simulink model "KvadroModel"  (R2013a)
settings: Solver=ode45  StartTime=0.0  StopTime=60  RelTol=1e-3
libraries: aerolibfltsims x2, vrlib x1, aerolib6dof2 x1, aerolibutil x1
settings Model: Creator=Mirag_000  LastModifiedBy=Mirag_000
settings DataIOCC: SignalLoggingSaveFormat=ModelDataLogs
settings DebuggingCC: MultiTaskDSMMsg=warning  MultiTaskCondExecSysMsg=none  StrictBusMsg=None
settings RTWCC: IncludeERTFirstTime=on

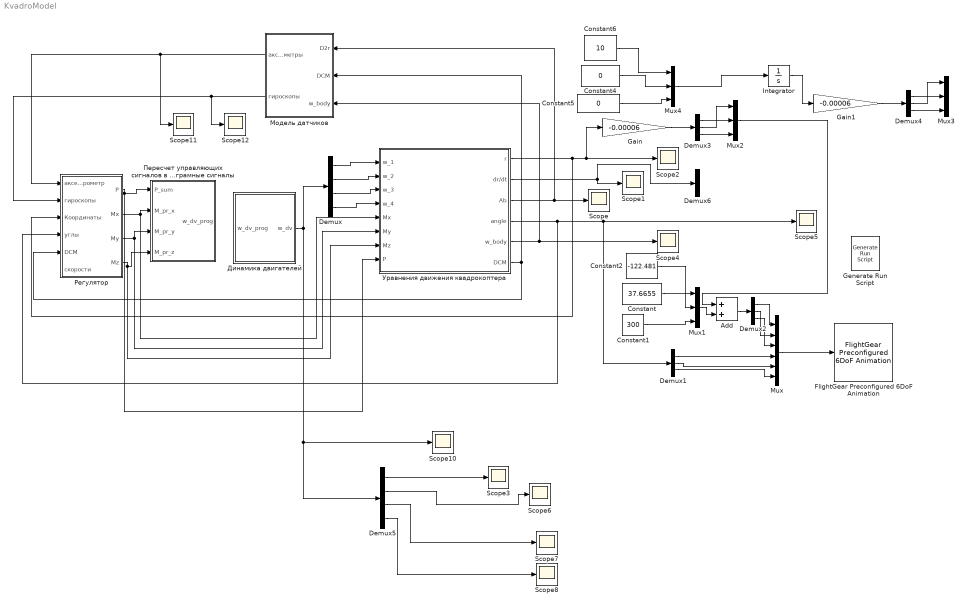
== system KvadroModel ==
  Add : Sum
  Constant : Constant  Value=37.6655
  Constant1 : Constant  Value=300
  Constant2 : Constant  Value=-122.481
  Constant4 : Constant  Value=0
  Constant5 : Constant  Value=0
  Constant6 : Constant  Value=10
  Demux : Demux
  Demux{1..4,6} (5 alike) : Demux  Outputs=3
  Demux5 : Demux
  FlightGear Preconfigured 6DoF Animation : aerolibfltsims/FlightGear Preconfigured 6DoF Animation  xFlightGearVersion=v2.8  DestinationIpAddress=127.0.0.1  DestinationPort=5502  SampleTime=1/30
  Gain : Gain  Gain=-0.00006
  Gain1 : Gain  Gain=-0.00006
  Generate Run Script : aerolibfltsims/Generate Run Script  OutputFileName=I:\Program Files\FlightGear\runfg.bat  FlightGearBaseDirectory=I:\Program Files\FlightGear  GeometryModelName=arducopter  DestinationPort=5502  OriginAddress=127.0.0.1  OriginPort=5505  LocalAddress=127.0.0.1  AirportId=KSFO  RunwayId=10L  InitialAltitude=7224  InitialHeading=113  OffsetDistance=4.72  OffsetAzimuth=0  GenerateFile=off  Architecture=Default  dataFlow=Send
  Integrator : Integrator
  Mux : Mux  Inputs=6
  Mux{1..4} (4 alike) : Mux  Inputs=3
  Scope{,1..8,10..12} (12 alike) : Scope
      Scope settings: TimeRange=60  YMin=-10  YMax=25
      Scope1 settings: YMin=-40  YMax=15  SaveName=ScopeData4
      Scope10 settings: YMin=1.5  YMax=3.75  SaveName=ScopeData12
      Scope11 settings: SaveName=ScopeData14
      Scope12 settings: SaveName=ScopeData15
      Scope2 settings: YMin=-80  YMax=90  SaveName=ScopeData5
      Scope3 settings: YMin=5.745  YMax=5.805  SaveName=ScopeData37
      Scope4 settings: YMin=-0.2  YMax=0.025  SaveName=ScopeData6
      Scope5 settings: YMin=-1.4  YMax=0.2  SaveName=ScopeData7
      Scope6 settings: YMin=5.73  YMax=5.82  SaveName=ScopeData38
      Scope7 settings: YMin=1.6525  YMax=1.675  SaveName=ScopeData46
      Scope8 settings: YMin=1.5  YMax=3.75  SaveName=ScopeData47
  Динамика двигателей : Subsystem
  Модель датчиков : Subsystem
  Пересчет управляющих сигналов в програмные сигналы : Subsystem
  Регулятор : Subsystem
  Уравнения движения квадрокоптера : Subsystem
  wires:
  Уравнения движения квадрокоптера/3(Ab) -> Scope/1, Модель датчиков/1(D2r)
  Уравнения движения квадрокоптера/2(dr/dt) -> Scope1/1, Demux6/1
  Уравнения движения квадрокоптера/1(r) -> Регулятор/3(Координаты), Gain/1, Scope2/1
  Уравнения движения квадрокоптера/5(w_body) -> Scope4/1, Модель датчиков/3(w_body)
  Уравнения движения квадрокоптера/4(angle) -> Регулятор/4(углы), Demux1/1, Scope5/1
  Demux/1 -> Уравнения движения квадрокоптера/1(w_1)
  Demux/2 -> Уравнения движения квадрокоптера/2(w_2)
  Demux/3 -> Уравнения движения квадрокоптера/3(w_3)
  Demux/4 -> Уравнения движения квадрокоптера/4(w_4)
  Динамика двигателей/1(w_dv) -> Demux5/1, Scope10/1, Demux/1
  Регулятор/1(P) -> Пересчет управляющих сигналов в програмные сигналы/1(P_sum), Уравнения движения квадрокоптера/8(P)
  Модель датчиков/1(акселерометры) -> Scope11/1, Регулятор/1(акселерометр)
  Модель датчиков/2(гироскопы) -> Scope12/1, Регулятор/2(гироскопы)
  Регулятор/2(Mx) -> Уравнения движения квадрокоптера/5(Mx), Пересчет управляющих сигналов в програмные сигналы/2(M_pr_x)
  Регулятор/3(My) -> Уравнения движения квадрокоптера/6(My), Пересчет управляющих сигналов в програмные сигналы/3(M_pr_y)
  Уравнения движения квадрокоптера/6("DCM ") -> Регулятор/5(DCM), Модель датчиков/2(DCM)
  Demux1/3 -> Mux/6
  Demux1/2 -> Mux/5
  Demux1/1 -> Mux/4
  Mux/1 -> FlightGear Preconfigured 6DoF Animation/1
  Constant2/1 -> Mux1/1
  Constant/1 -> Mux1/2
  Constant1/1 -> Mux1/3
  Mux1/1 -> Add/2
  Add/1 -> Demux2/1
  Demux2/3 -> Mux/3
  Demux2/2 -> Mux/2
  Demux2/1 -> Mux/1
  Gain/1 -> Demux3/1
  Demux3/3 -> Mux2/3
  Gain1/1 -> Demux4/1
  Demux4/3 -> Mux3/3
  Demux4/2 -> Mux3/1
  Demux4/1 -> Mux3/2
  Integrator/1 -> Gain1/1
  Constant5/1 -> Mux4/3
  Mux4/1 -> Integrator/1
  Constant6/1 -> Mux4/1
  Constant4/1 -> Mux4/2
  Mux2/1 -> Add/1
  Demux3/1 -> Mux2/2
  Demux3/2 -> Mux2/1
  Demux5/1 -> Scope3/1
  Demux5/2 -> Scope6/1
  Demux5/3 -> Scope7/1
  Demux5/4 -> Scope8/1
  Регулятор/4(Mz) -> Уравнения движения квадрокоптера/7(Mz), Пересчет управляющих сигналов в програмные сигналы/4(M_pr_z)

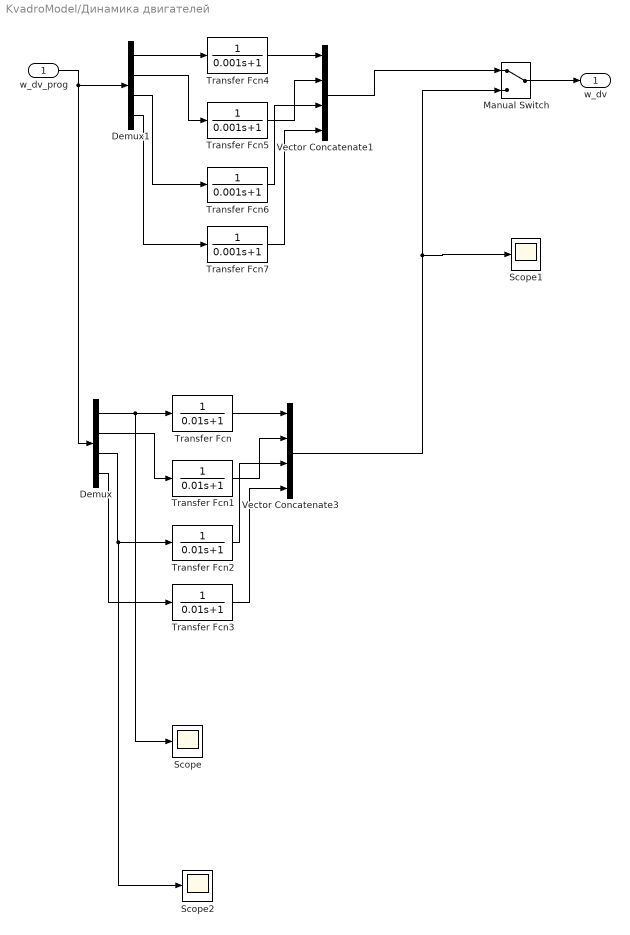
== system KvadroModel/Динамика двигателей ==
  w_dv_prog : Inport
  Demux : Demux
  Demux1 : Demux
  Manual Switch : ManualSwitch
  Scope : Scope
      settings: TimeRange=60  YMin=1.6595  YMax=1.668  SaveName=ScopeData39
  Scope1 : Scope
      settings: YMin=1.655  YMax=1.675  SaveName=ScopeData42
  Scope2 : Scope
      settings: YMin=1.6595  YMax=1.668  SaveName=ScopeData50
  Transfer Fcn{,1..3} (4 alike) : TransferFcn  Denominator=[0.01 1]
  Transfer Fcn{4..7} (4 alike) : TransferFcn  Denominator=[0.001 1]
  Vector Concatenate1 : Concatenate  NumInputs=4
  Vector Concatenate3 : Concatenate  NumInputs=4
  w_dv : Outport
  wires:
  Transfer Fcn1/1 -> Vector Concatenate3/2
  Transfer Fcn2/1 -> Vector Concatenate3/3
  Transfer Fcn3/1 -> Vector Concatenate3/4
  Vector Concatenate3/1 -> Scope1/1, Manual Switch/2
  Demux/1 -> Scope/1, Transfer Fcn/1
  Transfer Fcn/1 -> Vector Concatenate3/1
  Demux/2 -> Transfer Fcn1/1
  Demux/3 -> Scope2/1, Transfer Fcn2/1
  Demux/4 -> Transfer Fcn3/1
  Manual Switch/1 -> w_dv/1
  w_dv_prog/1 -> Demux/1, Demux1/1
  Transfer Fcn5/1 -> Vector Concatenate1/2
  Transfer Fcn6/1 -> Vector Concatenate1/3
  Transfer Fcn7/1 -> Vector Concatenate1/4
  Demux1/1 -> Transfer Fcn4/1
  Transfer Fcn4/1 -> Vector Concatenate1/1
  Demux1/2 -> Transfer Fcn5/1
  Demux1/3 -> Transfer Fcn6/1
  Demux1/4 -> Transfer Fcn7/1
  Vector Concatenate1/1 -> Manual Switch/1

== system KvadroModel/Модель датчиков ==
  D2r : Inport
  DCM : Inport  Port=2
  w_body : Inport  Port=3
  Add : Sum  Inputs=+-
  Constant : Constant  Value=[0 0 -9.81]
  Product : Product  Multiplication=Matrix(*)  RndMeth=Zero
  Scope : Scope
      settings: SaveName=ScopeData24
  акселерометры : Outport
  гироскопы : Outport  Port=2
  wires:
  D2r/1 -> Add/1
  w_body/1 -> Scope/1, гироскопы/1
  DCM/1 -> Product/1
  Constant/1 -> Product/2
  Product/1 -> Add/2
  Add/1 -> акселерометры/1

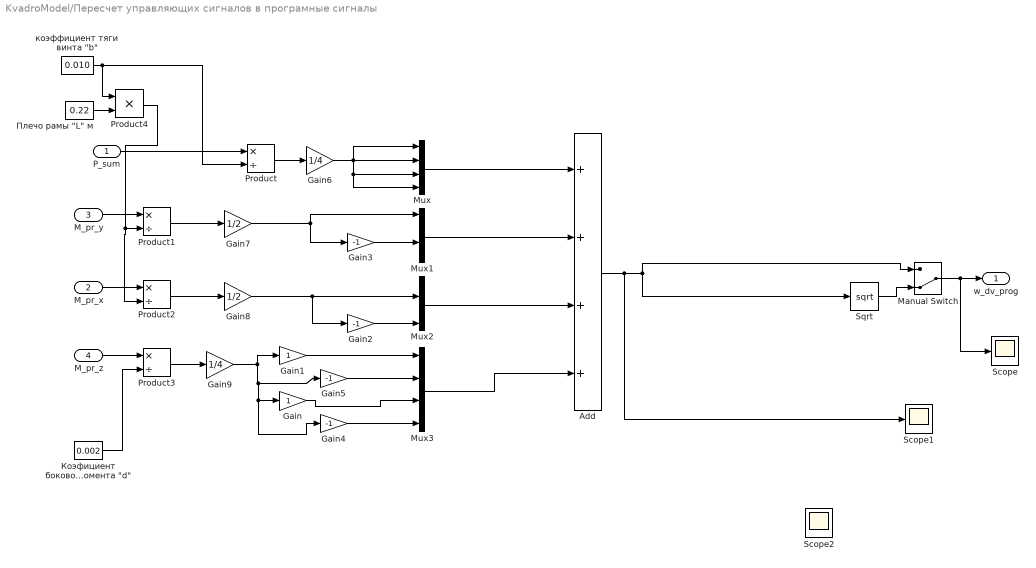
== system KvadroModel/Пересчет управляющих сигналов в програмные сигналы ==
  P_sum : Inport
  M_pr_x : Inport  Port=2
  M_pr_y : Inport  Port=3
  M_pr_z : Inport  Port=4
  Add : Sum  Inputs=++++
  Gain : Gain
  Gain1 : Gain
  Gain{2..5} (4 alike) : Gain  Gain=-1
  Gain6 : Gain  Gain=1/4
  Gain7 : Gain  Gain=1/2
  Gain8 : Gain  Gain=1/2
  Gain9 : Gain  Gain=1/4
  Manual Switch : ManualSwitch  CurrentSetting=0
  Mux{,1..3} (4 alike) : Mux
  Product{,1..3} (4 alike) : Product  Inputs=*/
  Product4 : Product
  Scope : Scope
      settings: YMin=1.6575  YMax=1.6775  SaveName=ScopeData20
  Scope1 : Scope
      settings: YMin=60  YMax=180  SaveName=ScopeData34
  Scope2 : Scope
      settings: YMin=0.07  YMax=0.1025  SaveName=ScopeData44
  Sqrt : Sqrt  SaturateOnIntegerOverflow=on
  "Коэфициент бокового момента \"d\"" : Constant  Value=0.002
  "Плечо рамы \"L\" м" : Constant  Value=0.22
  "коэффициент тяги винта \"b\"" : Constant  Value=0.010
  w_dv_prog : Outport
  wires:
  Gain/1 -> Mux3/3
  Gain1/1 -> Mux3/1
  Product3/1 -> Gain9/1
  Product2/1 -> Gain8/1
  Gain2/1 -> Mux2/4
  Gain3/1 -> Mux1/3
  Product1/1 -> Gain7/1
  Product/1 -> Gain6/1
  Mux2/1 -> Add/3
  Mux1/1 -> Add/2
  Mux/1 -> Add/1
  Mux3/1 -> Add/4
  Gain5/1 -> Mux3/2
  Gain4/1 -> Mux3/4
  Manual Switch/1 -> w_dv_prog/1, Scope/1
  Sqrt/1 -> Manual Switch/2
  Add/1 -> Scope1/1, Manual Switch/1, Sqrt/1
  P_sum/1 -> Product/1
  M_pr_y/1 -> Product1/1
  M_pr_x/1 -> Product2/1
  M_pr_z/1 -> Product3/1
  "Коэфициент бокового момента \"d\""/1 -> Product3/2
  "Плечо рамы \"L\" м"/1 -> Product4/2
  "коэффициент тяги винта \"b\""/1 -> Product/2, Product4/1
  Product4/1 -> Product2/2, Product1/2
  Gain6/1 -> Mux/4, Mux/3, Mux/1, Mux/2
  Gain7/1 -> Gain3/1, Mux1/1
  Gain8/1 -> Gain2/1, Mux2/2
  Gain9/1 -> Gain1/1, Gain4/1, Gain/1, Gain5/1

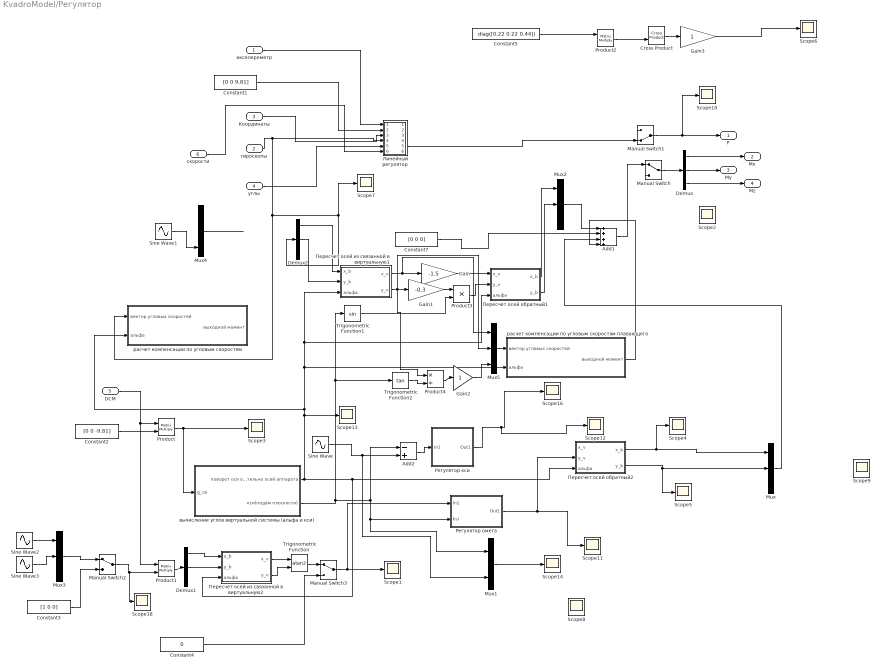
== system KvadroModel/Регулятор ==
  акселерометр : Inport
  гироскопы : Inport  Port=2
  Координаты : Inport  Port=3
  углы : Inport  Port=4
  DCM : Inport  Port=5
  скорости : Inport  Port=6
  Add1 : Sum  Inputs=++++
  Add2 : Sum  Inputs=-+
  Constant1 : Constant  Value=[0 0 9.81]
  Constant2 : Constant  Value=[0 0 -9.81]
  Constant3 : Constant  Value=[1 0 0]
  Constant4 : Constant  Value=0
  Constant5 : Constant  Value=diag([0.22 0.22 0.44])
  Constant7 : Constant  Value=[0 0 0]
  Cross Product : vrlib/Utilities/Cross Product
  Demux : Demux  Outputs=3
  Demux1 : Demux  Outputs=3
  Demux2 : Demux  Outputs=3
  Gain : Gain  Gain=-1.5
  Gain1 : Gain  Gain=-0.3
  Gain2 : Gain
  Gain3 : Gain
  Manual Switch : ManualSwitch
  Manual Switch1 : ManualSwitch  CurrentSetting=0
  Manual Switch2 : ManualSwitch
  Manual Switch3 : ManualSwitch
  Mux{,2..5} (5 alike) : Mux  Inputs=3
  Mux1 : Mux  Inputs=2
  Product : Product  Multiplication=Matrix(*)
  Product1 : Product  Multiplication=Matrix(*)
  Product2 : Product  Multiplication=Matrix(*)
  Product3 : Product  Inputs=**
  Product4 : Product  Inputs=*/
  Scope{1..14,16,18} (16 alike) : Scope
      Scope1 settings: TimeRange=10  YMin=-3.5  YMax=3.5
      Scope10 settings: YMin=4.66  YMax=4.78  SaveName=ScopeData27
      Scope11 settings: TimeRange=10  YMin=-0.275  YMax=0.125  SaveName=ScopeData57
      Scope12 settings: YMin=1.875  YMax=2.175  SaveName=ScopeData63
      Scope13 settings: TimeRange=10  YMin=-0.827297  YMax=-0.748507  SaveName=ScopeData49
      Scope14 settings: TimeRange=1  YMin=0.275  YMax=0.5  SaveName=ScopeData51
      Scope16 settings: TimeRange=20  YMin=-1.5  YMax=2  SaveName=ScopeData68
      Scope18 settings: TimeRange=20  YMin=0.2  YMax=1.5  SaveName=ScopeData48
      Scope2 settings: YMin=-0.0025  YMax=0.025  SaveName=ScopeData3
      Scope3 settings: YMin=-10  YMax=10  SaveName=ScopeData16
      Scope4 settings: YMin=-0.004  YMax=0.006  SaveName=ScopeData17
      Scope5 settings: TimeRange=10  YMin=0.0122457  YMax=0.0135347  SaveName=ScopeData22
      Scope6 settings: YMin=-0.001  YMax=0.001  SaveName=ScopeData32
      Scope7 settings: YMin=-1  YMax=1.25  SaveName=ScopeData35
      Scope8 settings: TimeRange=20  YMin=0.1  YMax=0.8  SaveName=ScopeData56
      Scope9 settings: TimeRange=20  YMin=-0.025  YMax=0.35  SaveName=ScopeData26
  Sine Wave : Sin  Amplitude=0  Bias=0.5  Frequency=0.4  SampleTime=0
  Sine Wave1 : Sin  Amplitude=0  Frequency=0.07  SampleTime=0
  Sine Wave2 : Sin  SampleTime=0
  Sine Wave3 : Sin  Phase=3.14/2  SampleTime=0
  Trigonometric Function : Trigonometry  Operator=atan2
  Trigonometric Function1 : Trigonometry
  Trigonometric Function2 : Trigonometry  Operator=tan
  Линейный регулятор : Subsystem
  Пересчет осей из связанной в виртуальную1 : Subsystem
  Пересчет осей из связанной в виртуальную2 : Subsystem
  Пересчет осей обратный1 : Subsystem
  Пересчет осей обратный2 : Subsystem
  Регулятор кси : Subsystem
  Регулятор омега : Subsystem
  вычисление углов виртуальной системы (альфа и кси) : Subsystem
  расчет компенсации по угловым скоростям : Subsystem
  расчет компенсации по угловым скоростям плавающего : Subsystem
  P : Outport
  Mx : Outport  Port=2
  My : Outport  Port=3
  Mz : Outport  Port=4
  wires:
  Demux/1 -> Mx/1
  Demux/2 -> My/1
  Demux/3 -> Mz/1
  Manual Switch/1 -> Demux/1
  Manual Switch1/1 -> Scope10/1, P/1
  Координаты/1 -> Линейный регулятор/3(In3)
  Линейный регулятор/5(Out5) -> Manual Switch1/2
  углы/1 -> Линейный регулятор/5(In5)
  Constant2/1 -> Product/2
  DCM/1 -> Product1/1, Product/1
  Product/1 -> Scope3/1, вычисление углов виртуальной системы (альфа и кси)/1(g_св)
  Constant1/1 -> Линейный регулятор/2(In2)
  акселерометр/1 -> Линейный регулятор/1(In1)
  гироскопы/1 -> расчет компенсации по угловым скоростям/1(вектор угловых скоростей), Scope7/1, Demux2/1, Линейный регулятор/4(In4)
  Constant5/1 -> Product2/1
  Product2/1 -> Cross Product/2
  Cross Product/1 -> Gain3/1
  Gain3/1 -> Scope6/1
  Sine Wave/1 -> Add2/2, Mux1/2
  Mux1/1 -> Scope14/1
  Product1/1 -> Demux1/1
  Demux1/2 -> Пересчет осей из связанной в виртуальную2/2(y_b)
  Demux1/1 -> Пересчет осей из связанной в виртуальную2/1(x_b)
  Пересчет осей из связанной в виртуальную2/1(x_v) -> Trigonometric Function/1
  Пересчет осей из связанной в виртуальную2/2(y_v) -> Trigonometric Function/2
  Add2/1 -> Регулятор кси/1(In1)
  вычисление углов виртуальной системы (альфа и кси)/2(кси(подём плоскости)) -> Trigonometric Function2/1, Trigonometric Function1/1, Add2/1, Регулятор омега/2(ksi), Mux1/1
  Sine Wave2/1 -> Mux3/1
  Sine Wave3/1 -> Mux3/2
  скорости/1 -> Линейный регулятор/6(In6)
  Регулятор кси/1(Out1) -> Scope12/1, Scope16/1
  Mux4/1 -> ?
  Sine Wave1/1 -> Mux4/3
  Mux3/1 -> Manual Switch2/1
  Manual Switch2/1 -> Scope18/1, Product1/2
  Constant3/1 -> Manual Switch2/2
  Trigonometric Function/1 -> Manual Switch3/1
  Constant4/1 -> Manual Switch3/2
  Manual Switch3/1 -> Регулятор омега/1(In1), Scope1/1
  Регулятор омега/1(Out1) -> Пересчет осей обратный2/2(y_v), Scope11/1
  Demux2/1 -> Пересчет осей из связанной в виртуальную1/1(x_b)
  Пересчет осей из связанной в виртуальную1/1(x_v) -> Mux5/1, Gain/1
  Пересчет осей обратный2/1(x_b) -> Scope4/1, Mux/1
  Demux2/2 -> Пересчет осей из связанной в виртуальную1/2(y_b)
  Gain/1 -> Пересчет осей обратный1/1(x_v)
  Пересчет осей обратный1/1(x_b) -> Mux2/1
  Пересчет осей обратный1/2(y_b) -> Mux2/2
  Пересчет осей из связанной в виртуальную1/2(y_v) -> Product4/1, Mux5/2, Gain1/1
  вычисление углов виртуальной системы (альфа и кси)/1(поворот оси относительно осей аппарата) -> Scope13/1, Пересчет осей обратный1/3(альфа), Пересчет осей из связанной в виртуальную1/3(альфа), расчет компенсации по угловым скоростям плавающего/2(альфа), расчет компенсации по угловым скоростям/2(альфа), Пересчет осей обратный2/3(альфа), Пересчет осей из связанной в виртуальную2/3(альфа)
  Trigonometric Function1/1 -> Product3/2
  Gain1/1 -> Product3/1
  Add1/1 -> Manual Switch/1
  Constant7/1 -> Add1/2
  Mux/1 -> Add1/3
  Mux2/1 -> Add1/1
  Пересчет осей обратный2/2(y_b) -> Mux/2, Scope5/1
  Product3/1 -> Пересчет осей обратный1/2(y_v)
  Mux5/1 -> расчет компенсации по угловым скоростям плавающего/1(вектор угловых скоростей)
  Trigonometric Function2/1 -> Product4/2
  Product4/1 -> Gain2/1
  Gain2/1 -> Mux5/3
  расчет компенсации по угловым скоростям плавающего/1(выходной момент) -> Add1/4

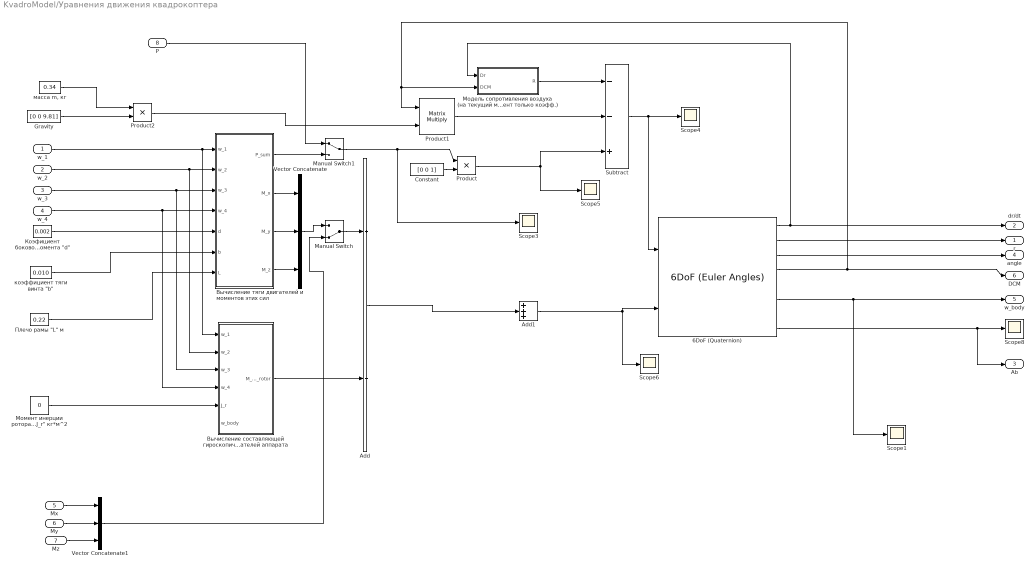
== system KvadroModel/Уравнения движения квадрокоптера ==
  w_1 : Inport
  w_2 : Inport  Port=2
  w_3 : Inport  Port=3
  w_4 : Inport  Port=4
  Mx : Inport  Port=5
  My : Inport  Port=6
  Mz : Inport  Port=7
  P : Inport  Port=8
  6DoF (Quaternion) : aerolib6dof2/6DoF (Euler Angles)  units=Metric (MKS)  mtype=Fixed  rep=Quaternion  xme_0=[0 0 0]  Vm_0=[0 0 0]  eul_0=[0.3 0 0]  pm_0=[0 0 0]  mass_0=0.340  mass_e=0  mass_f=0  inertia=diag([0.22 0.22 0.44])  inertia_e=eye(3)  inertia_f=eye(3)  k_quat=1.0
  Add : Sum  Inputs=+-
  Add1 : Sum  Inputs=+++
  Constant : Constant  Value=[0 0 1]
  Gravity : Constant  Value=[0 0 9.81]
  Manual Switch : ManualSwitch  CurrentSetting=0
  Manual Switch1 : ManualSwitch
  Product : Product
  Product1 : Product  Multiplication=Matrix(*)  RndMeth=Zero
  Product2 : Product  RndMeth=Zero
  Scope{1,3..6,8} (6 alike) : Scope
      Scope1 settings: YMin=-0.05  YMax=0.7  SaveName=ScopeData36
      Scope3 settings: YMin=0  YMax=60  SaveName=ScopeData41
      Scope4 settings: SaveName=ScopeData18
      Scope5 settings: SaveName=ScopeData19
      Scope6 settings: TimeRange=40  YMin=-0.01  YMax=0.1  SaveName=ScopeData21
      Scope8 settings: SaveName=ScopeData23
  Subtract : Sum  Inputs=--+
  Vector Concatenate : Concatenate  NumInputs=3
  Vector Concatenate1 : Concatenate  NumInputs=3
  Вычисление составляющей гироскопического момента роторов двигателей аппарата : Subsystem
  Вычисление тяги двигателей и моментов этих сил : Subsystem
  "Коэфициент бокового момента \"d\"" : Constant  Value=0.002
  Модель сопротивления воздуха (на текущий момент только коэфф.) : Subsystem
  "Момент инерции ротора \"J_r\" кг*м^2" : Constant  Value=0
  "Плечо рамы \"L\" м" : Constant  Value=0.22
  "коэффициент тяги винта \"b\"" : Constant  Value=0.010
  "масса m, кг" : Constant  Value=0.34
  r : Outport
  dr/dt : Outport  Port=2
  Ab : Outport  Port=3
  angle : Outport  Port=4
  w_body : Outport  Port=5
  "DCM " : Outport  Port=6
  wires:
  w_1/1 -> Вычисление составляющей гироскопического момента роторов двигателей аппарата/1(w_1), Вычисление тяги двигателей и моментов этих сил/1(w_1)
  w_2/1 -> Вычисление составляющей гироскопического момента роторов двигателей аппарата/2(w_2), Вычисление тяги двигателей и моментов этих сил/2(w_2)
  w_3/1 -> Вычисление тяги двигателей и моментов этих сил/3(w_3), Вычисление составляющей гироскопического момента роторов двигателей аппарата/3(w_3)
  w_4/1 -> Вычисление составляющей гироскопического момента роторов двигателей аппарата/4(w_4), Вычисление тяги двигателей и моментов этих сил/4(w_4)
  "Коэфициент бокового момента \"d\""/1 -> Вычисление тяги двигателей и моментов этих сил/5(d)
  "коэффициент тяги винта \"b\""/1 -> Вычисление тяги двигателей и моментов этих сил/6(b)
  "Плечо рамы \"L\" м"/1 -> Вычисление тяги двигателей и моментов этих сил/7(L)
  Вычисление тяги двигателей и моментов этих сил/2(M_x) -> Vector Concatenate/1
  Вычисление тяги двигателей и моментов этих сил/3(M_y) -> Vector Concatenate/2
  Вычисление тяги двигателей и моментов этих сил/4(M_z) -> Vector Concatenate/3
  "Момент инерции ротора \"J_r\" кг*м^2"/1 -> Вычисление составляющей гироскопического момента роторов двигателей аппарата/5(J_r)
  Вычисление составляющей гироскопического момента роторов двигателей аппарата/1(M_gyr_rotor) -> Add/2
  Constant/1 -> Product/2
  "масса m, кг"/1 -> Product2/1
  6DoF (Quaternion)/2 -> r/1
  Модель сопротивления воздуха (на текущий момент только коэфф.)/1(R) -> Subtract/1
  Gravity/1 -> Product2/2
  Add1/1 -> Scope6/1, 6DoF (Quaternion)/2
  6DoF (Quaternion)/3 -> angle/1
  6DoF (Quaternion)/4 -> "DCM "/1, Модель сопротивления воздуха (на текущий момент только коэфф.)/2(DCM), Product1/1
  Product2/1 -> Product1/2
  Product1/1 -> Subtract/2
  Subtract/1 -> 6DoF (Quaternion)/1, Scope4/1
  Product/1 -> Scope5/1, Subtract/3
  6DoF (Quaternion)/8 -> Ab/1, Scope8/1
  6DoF (Quaternion)/1 -> Модель сопротивления воздуха (на текущий момент только коэфф.)/1(Dr), dr/dt/1
  6DoF (Quaternion)/6 -> Scope1/1, w_body/1
  My/1 -> Vector Concatenate1/2
  Mx/1 -> Vector Concatenate1/1
  Mz/1 -> Vector Concatenate1/3
  Manual Switch/1 -> Add/1
  Vector Concatenate/1 -> Manual Switch/1
  Vector Concatenate1/1 -> Manual Switch/2
  Вычисление тяги двигателей и моментов этих сил/1(P_sum) -> Manual Switch1/2
  P/1 -> Manual Switch1/1
  Manual Switch1/1 -> Scope3/1, Product/1
  Add/1 -> Add1/2

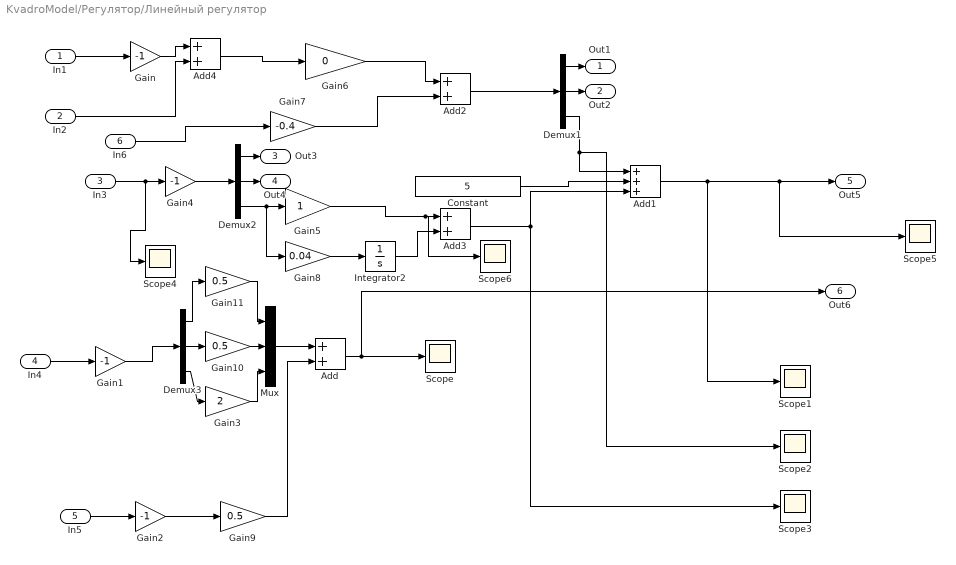
== system KvadroModel/Регулятор/Линейный регулятор ==
  In1 : Inport
  In2 : Inport  Port=2
  In3 : Inport  Port=3
  In4 : Inport  Port=4
  In5 : Inport  Port=5
  In6 : Inport  Port=6
  Add{,2..4} (4 alike) : Sum
  Add1 : Sum  Inputs=+++
  Constant : Constant  Value=5
  Demux1 : Demux  Outputs=3
  Demux2 : Demux  Outputs=3
  Demux3 : Demux  Outputs=3
  Gain{,1..2,4} (4 alike) : Gain  Gain=-1
  Gain10 : Gain  Gain=0.5
  Gain11 : Gain  Gain=0.5
  Gain3 : Gain  Gain=2
  Gain5 : Gain
  Gain6 : Gain  Gain=0
  Gain7 : Gain  Gain=-0.4
  Gain8 : Gain  Gain=0.04
  Gain9 : Gain  Gain=0.5
  Integrator2 : Integrator
  Mux : Mux  Inputs=3
  Scope{,1..6} (7 alike) : Scope
      Scope settings: YMin=-0.002  YMax=0.008  SaveName=ScopeData13
      Scope1 settings: SaveName=ScopeData28
      Scope2 settings: SaveName=ScopeData29
      Scope3 settings: SaveName=ScopeData30
      Scope4 settings: SaveName=ScopeData31
      Scope5 settings: YMin=7  YMax=21  SaveName=ScopeData40
      Scope6 settings: YMin=-35  YMax=0  SaveName=ScopeData52
  Out1 : Outport
  Out2 : Outport  Port=2
  Out3 : Outport  Port=3
  Out4 : Outport  Port=4
  Out5 : Outport  Port=5
  Out6 : Outport  Port=6
  wires:
  Gain7/1 -> Add2/2
  In3/1 -> Scope4/1, Gain4/1
  Demux1/3 -> Add1/1, Scope2/1
  Demux2/3 -> Gain8/1, Gain5/1
  Constant/1 -> Add1/2
  Gain4/1 -> Demux2/1
  Add/1 -> Out6/1, Scope/1
  In1/1 -> Gain/1
  In4/1 -> Gain1/1
  In2/1 -> Add4/2
  Gain/1 -> Add4/1
  Gain6/1 -> Add2/1
  Add3/1 -> Scope3/1, Add1/3
  Add2/1 -> Demux1/1
  Integrator2/1 -> Add3/2
  Gain5/1 -> Scope6/1, Add3/1
  Add1/1 -> Scope1/1, Scope5/1, Out5/1
  Gain8/1 -> Integrator2/1
  Demux2/1 -> Out3/1
  Demux2/2 -> Out4/1
  Demux1/2 -> Out2/1
  Demux1/1 -> Out1/1
  Gain9/1 -> Add/2
  In5/1 -> Gain2/1
  Gain2/1 -> Gain9/1
  Gain1/1 -> Demux3/1
  Demux3/3 -> Gain3/1
  Demux3/2 -> Gain10/1
  Demux3/1 -> Gain11/1
  Gain3/1 -> Mux/3
  Gain10/1 -> Mux/2
  Gain11/1 -> Mux/1
  Mux/1 -> Add/1
  Add4/1 -> Gain6/1
  In6/1 -> Gain7/1

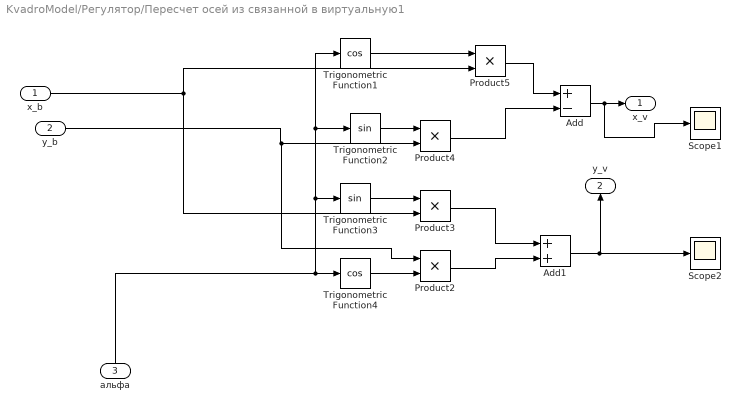
== system KvadroModel/Регулятор/Пересчет осей из связанной в виртуальную1 ==
  x_b : Inport
  y_b : Inport  Port=2
  альфа : Inport  Port=3
  Add : Sum  Inputs=+-
  Add1 : Sum
  Product{2..5} (4 alike) : Product
  Scope1 : Scope
      settings: YMin=-3.5  YMax=3.5  SaveName=ScopeData10
  Scope2 : Scope
      settings: YMin=-3.5  YMax=3.5  SaveName=ScopeData11
  Trigonometric Function1 : Trigonometry  Operator=cos
  Trigonometric Function2 : Trigonometry
  Trigonometric Function3 : Trigonometry
  Trigonometric Function4 : Trigonometry  Operator=cos
  x_v : Outport
  y_v : Outport  Port=2
  wires:
  Trigonometric Function4/1 -> Product2/2
  Trigonometric Function3/1 -> Product3/1
  Trigonometric Function2/1 -> Product4/1
  y_b/1 -> Product2/1, Product4/2
  Trigonometric Function1/1 -> Product5/1
  альфа/1 -> Trigonometric Function4/1, Trigonometric Function3/1, Trigonometric Function2/1, Trigonometric Function1/1
  Product5/1 -> Add/1
  Product4/1 -> Add/2
  Product3/1 -> Add1/1
  Product2/1 -> Add1/2
  Add1/1 -> Scope2/1, y_v/1
  Add/1 -> Scope1/1, x_v/1
  x_b/1 -> Product5/2, Product3/2

== system KvadroModel/Регулятор/Пересчет осей из связанной в виртуальную2 ==
  x_b : Inport
  y_b : Inport  Port=2
  альфа : Inport  Port=3
  Add : Sum  Inputs=+-
  Add1 : Sum
  Product{2..5} (4 alike) : Product
  Scope1 : Scope
      settings: YMin=-3.5  YMax=3.5  SaveName=ScopeData10
  Scope2 : Scope
      settings: YMin=-3.5  YMax=3.5  SaveName=ScopeData11
  Trigonometric Function1 : Trigonometry  Operator=cos
  Trigonometric Function2 : Trigonometry
  Trigonometric Function3 : Trigonometry
  Trigonometric Function4 : Trigonometry  Operator=cos
  x_v : Outport
  y_v : Outport  Port=2
  wires:
  Trigonometric Function4/1 -> Product2/2
  Trigonometric Function3/1 -> Product3/1
  Trigonometric Function2/1 -> Product4/1
  y_b/1 -> Product2/1, Product4/2
  Trigonometric Function1/1 -> Product5/1
  альфа/1 -> Trigonometric Function4/1, Trigonometric Function3/1, Trigonometric Function2/1, Trigonometric Function1/1
  Product5/1 -> Add/1
  Product4/1 -> Add/2
  Product3/1 -> Add1/1
  Product2/1 -> Add1/2
  Add1/1 -> Scope2/1, y_v/1
  Add/1 -> Scope1/1, x_v/1
  x_b/1 -> Product5/2, Product3/2

== system KvadroModel/Регулятор/Пересчет осей обратный1 ==
  x_v : Inport
  y_v : Inport  Port=2
  альфа : Inport  Port=3
  Add : Sum
  Add1 : Sum  Inputs=-+
  Product{2..5} (4 alike) : Product
  Scope1 : Scope
      settings: YMin=-3.5  YMax=3.5  SaveName=ScopeData10
  Scope2 : Scope
      settings: YMin=-3.5  YMax=3.5  SaveName=ScopeData11
  Trigonometric Function1 : Trigonometry  Operator=cos
  Trigonometric Function2 : Trigonometry
  Trigonometric Function3 : Trigonometry
  Trigonometric Function4 : Trigonometry  Operator=cos
  x_b : Outport
  y_b : Outport  Port=2
  wires:
  Add1/1 -> Scope2/1, y_b/1
  Add/1 -> Scope1/1, x_b/1
  Trigonometric Function4/1 -> Product2/2
  Trigonometric Function3/1 -> Product3/1
  Trigonometric Function2/1 -> Product4/1
  y_v/1 -> Product4/2, Product2/1
  Trigonometric Function1/1 -> Product5/1
  альфа/1 -> Trigonometric Function2/1, Trigonometric Function1/1, Trigonometric Function3/1, Trigonometric Function4/1
  Product5/1 -> Add/1
  Product4/1 -> Add/2
  Product3/1 -> Add1/1
  Product2/1 -> Add1/2
  x_v/1 -> Product3/2, Product5/2

== system KvadroModel/Регулятор/Пересчет осей обратный2 ==
  x_v : Inport
  y_v : Inport  Port=2
  альфа : Inport  Port=3
  Add : Sum
  Add1 : Sum  Inputs=-+
  Product{2..5} (4 alike) : Product
  Scope1 : Scope
      settings: YMin=-3.5  YMax=3.5  SaveName=ScopeData10
  Scope2 : Scope
      settings: YMin=-3.5  YMax=3.5  SaveName=ScopeData11
  Trigonometric Function1 : Trigonometry  Operator=cos
  Trigonometric Function2 : Trigonometry
  Trigonometric Function3 : Trigonometry
  Trigonometric Function4 : Trigonometry  Operator=cos
  x_b : Outport
  y_b : Outport  Port=2
  wires:
  Add1/1 -> Scope2/1, y_b/1
  Add/1 -> Scope1/1, x_b/1
  Trigonometric Function4/1 -> Product2/2
  Trigonometric Function3/1 -> Product3/1
  Trigonometric Function2/1 -> Product4/1
  y_v/1 -> Product4/2, Product2/1
  Trigonometric Function1/1 -> Product5/1
  альфа/1 -> Trigonometric Function2/1, Trigonometric Function1/1, Trigonometric Function3/1, Trigonometric Function4/1
  Product5/1 -> Add/1
  Product4/1 -> Add/2
  Product3/1 -> Add1/1
  Product2/1 -> Add1/2
  x_v/1 -> Product3/2, Product5/2

== system KvadroModel/Регулятор/Регулятор кси ==
  In1 : Inport
  Gain1 : Gain
  Gain5 : Gain
  Gain6 : Gain  Gain=0.01
  Integrator2 : Integrator
  Scope1 : Scope
      settings: TimeRange=20  YMin=-0.08  YMax=-1.38778e-17  SaveName=ScopeData54
  Sum1 : Sum  Inputs=|++++
  Out1 : Outport
  wires:
  Gain1/1 -> Sum1/1
  In1/1 -> Gain5/1
  Sum1/1 -> Out1/1
  Gain6/1 -> Integrator2/1
  Integrator2/1 -> Scope1/1, Sum1/2
  Gain5/1 -> Gain6/1, Gain1/1

== system KvadroModel/Регулятор/Регулятор омега ==
  In1 : Inport
  ksi : Inport  Port=2
  Gain1 : Gain  Gain=0
  Gain2 : Gain  Gain=-1
  Gain6 : Gain  Gain=0.1
  Integrator : Integrator
  Product : Product  Inputs=**
  Scope : Scope
      settings: YMin=-0.0825  YMax=-0.0425  SaveName=ScopeData2
  Scope1 : Scope
      settings: YMin=0.0005  YMax=0.007  SaveName=ScopeData25
  Scope2 : Scope
      settings: YMin=0.00119  YMax=0.001265  SaveName=ScopeData33
  Sum : Sum  Inputs=|++
  Sum1 : Sum  Inputs=|+++
  Trigonometric Function : Trigonometry
  Out1 : Outport
  wires:
  Gain1/1 -> Integrator/1
  Gain6/1 -> Sum/1, Scope2/1
  Integrator/1 -> Sum/2
  Sum/1 -> Sum1/1
  Sum1/1 -> Product/2, Scope/1
  ksi/1 -> Trigonometric Function/1
  Gain2/1 -> Gain1/1, Gain6/1
  In1/1 -> Gain2/1
  Product/1 -> Scope1/1, Out1/1
  Trigonometric Function/1 -> Product/1

== system KvadroModel/Регулятор/вычисление углов виртуальной системы (альфа и кси) ==
  g_св : Inport
  Add : Sum
  Demux1 : Demux  Outputs=3
  Gain : Gain  Gain=-1
  Gain1 : Gain  Gain=-1
  Gain2 : Gain  Gain=-1
  Gain3 : Gain
  Product1 : Product  Inputs=*/
  Product2 : Product
  Product3 : Product
  Scope1 : Scope
      settings: TimeRange=20  YMin=-1.75  YMax=1.75  SaveName=ScopeData59
  Scope3 : Scope
      settings: TimeRange=20  YMin=-3.25  YMax=0  SaveName=ScopeData55
  Sqrt : Sqrt  SaturateOnIntegerOverflow=on
  Trigonometric Function : Trigonometry  Operator=atan2
  Trigonometric Function1 : Trigonometry  Operator=atan
  поворот оси относительно осей аппарата : Outport
  кси(подём плоскости) : Outport  Port=2
  wires:
  Product1/1 -> Trigonometric Function1/1
  g_св/1 -> Demux1/1
  Demux1/2 -> Product3/2, Product3/1, Gain/1
  Demux1/1 -> Product2/2, Product2/1, Gain2/1
  Product2/1 -> Add/1
  Product3/1 -> Add/2
  Add/1 -> Sqrt/1
  Trigonometric Function1/1 -> Gain1/1
  Trigonometric Function/1 -> Gain3/1, Scope3/1
  Gain1/1 -> Scope1/1, кси(подём плоскости)/1
  Gain3/1 -> поворот оси относительно осей аппарата/1
  Gain2/1 -> Trigonometric Function/1
  Gain/1 -> Trigonometric Function/2
  Sqrt/1 -> Product1/1
  Demux1/3 -> Product1/2

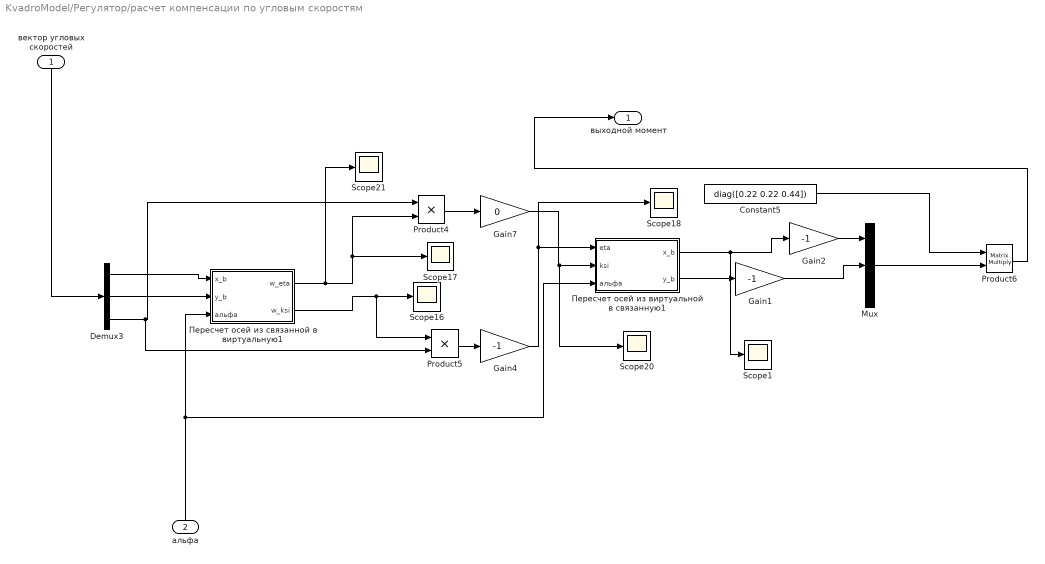
== system KvadroModel/Регулятор/расчет компенсации по угловым скоростям ==
  вектор угловых скоростей : Inport
  альфа : Inport  Port=2
  Constant5 : Constant  Value=diag([0.22 0.22 0.44])
  Demux3 : Demux  Outputs=3
  Gain1 : Gain  Gain=-1
  Gain2 : Gain  Gain=-1
  Gain4 : Gain  Gain=-1
  Gain7 : Gain  Gain=0
  Mux : Mux  Inputs=3
  Product4 : Product
  Product5 : Product
  Product6 : Product  Multiplication=Matrix(*)
  Scope{1,16..18,20..21} (6 alike) : Scope
      Scope1 settings: YMin=-0.02  YMax=0.015  SaveName=ScopeData58
      Scope16 settings: YMin=-0.00045  YMax=0.0002  SaveName=ScopeData65
      Scope17 settings: TimeRange=20  YMin=-0.015  YMax=0.015  SaveName=ScopeData66
      Scope18 settings: YMin=-0.01  YMax=0.1  SaveName=ScopeData67
      Scope20 settings: YMin=-0.5  YMax=0.5  SaveName=ScopeData69
      Scope21 settings: TimeRange=20  YMin=0.015  YMax=0.085  SaveName=ScopeData70
  Пересчет осей из виртуальной в связанную1 : Subsystem
  Пересчет осей из связанной в виртуальную1 : Subsystem
  выходной момент : Outport
  wires:
  Demux3/2 -> Пересчет осей из связанной в виртуальную1/2(y_b)
  Demux3/1 -> Пересчет осей из связанной в виртуальную1/1(x_b)
  Product5/1 -> Gain4/1
  Gain4/1 -> Пересчет осей из виртуальной в связанную1/1(eta), Scope18/1
  Product4/1 -> Gain7/1
  Gain7/1 -> Пересчет осей из виртуальной в связанную1/2(ksi), Scope20/1
  Пересчет осей из связанной в виртуальную1/2(w_ksi) -> Product5/1, Scope16/1
  Пересчет осей из связанной в виртуальную1/1(w_eta) -> Scope21/1, Product4/2, Scope17/1
  Product6/1 -> выходной момент/1
  Demux3/3 -> Product5/2, Product4/1
  альфа/1 -> Пересчет осей из виртуальной в связанную1/3(альфа), Пересчет осей из связанной в виртуальную1/3(альфа)
  вектор угловых скоростей/1 -> Demux3/1
  Mux/1 -> Product6/2
  Constant5/1 -> Product6/1
  Пересчет осей из виртуальной в связанную1/1(x_b) -> Scope1/1, Gain2/1
  Пересчет осей из виртуальной в связанную1/2(y_b) -> Gain1/1
  Gain2/1 -> Mux/1
  Gain1/1 -> Mux/2

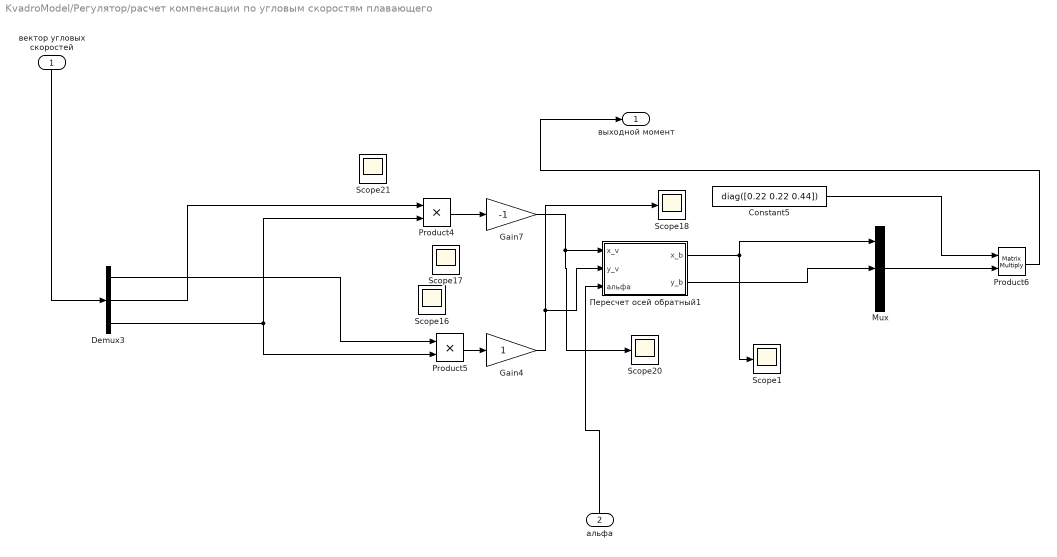
== system KvadroModel/Регулятор/расчет компенсации по угловым скоростям плавающего ==
  вектор угловых скоростей : Inport
  альфа : Inport  Port=2
  Constant5 : Constant  Value=diag([0.22 0.22 0.44])
  Demux3 : Demux  Outputs=3
  Gain4 : Gain
  Gain7 : Gain  Gain=-1
  Mux : Mux  Inputs=3
  Product4 : Product
  Product5 : Product
  Product6 : Product  Multiplication=Matrix(*)
  Scope{1,16..18,20..21} (6 alike) : Scope
      Scope1 settings: YMin=-0.02  YMax=0.015  SaveName=ScopeData58
      Scope16 settings: YMin=-0.00045  YMax=0.0002  SaveName=ScopeData65
      Scope17 settings: TimeRange=20  YMin=-0.015  YMax=0.015  SaveName=ScopeData66
      Scope18 settings: YMin=-0.01  YMax=0.1  SaveName=ScopeData67
      Scope20 settings: YMin=-0.5  YMax=0.5  SaveName=ScopeData69
      Scope21 settings: TimeRange=20  YMin=0.015  YMax=0.085  SaveName=ScopeData70
  Пересчет осей обратный1 : Subsystem
  выходной момент : Outport
  wires:
  Product5/1 -> Gain4/1
  Gain4/1 -> Пересчет осей обратный1/2(y_v), Scope18/1
  Product4/1 -> Gain7/1
  Gain7/1 -> Пересчет осей обратный1/1(x_v), Scope20/1
  Product6/1 -> выходной момент/1
  вектор угловых скоростей/1 -> Demux3/1
  Mux/1 -> Product6/2
  Constant5/1 -> Product6/1
  Пересчет осей обратный1/1(x_b) -> Mux/1, Scope1/1
  Пересчет осей обратный1/2(y_b) -> Mux/2
  альфа/1 -> Пересчет осей обратный1/3(альфа)
  Demux3/3 -> Product5/2, Product4/2
  Demux3/1 -> Product5/1
  Demux3/2 -> Product4/1

== system KvadroModel/Уравнения движения квадрокоптера/Вычисление составляющей гироскопического момента роторов двигателей аппарата ==
  w_1 : Inport
  w_2 : Inport  Port=2
  w_3 : Inport  Port=3
  w_4 : Inport  Port=4
  J_r : Inport  Port=5
  w_body : Inport  Port=6
  3x3 Cross Product : aerolibutil/3x3 Cross Product
  Add1 : Sum  Inputs=++--
  Constant5 : Constant  Value=[0 0 1]
  Product : Product
  Product1 : Product
  M_gyr_rotor : Outport
  wires:
  Add1/1 -> Product/1
  3x3 Cross Product/1 -> Product/2
  w_body/1 -> 3x3 Cross Product/1
  Constant5/1 -> 3x3 Cross Product/2
  J_r/1 -> Product1/2
  Product/1 -> Product1/1
  Product1/1 -> M_gyr_rotor/1
  w_2/1 -> Add1/3
  w_3/1 -> Add1/2
  w_1/1 -> Add1/1
  w_4/1 -> Add1/4

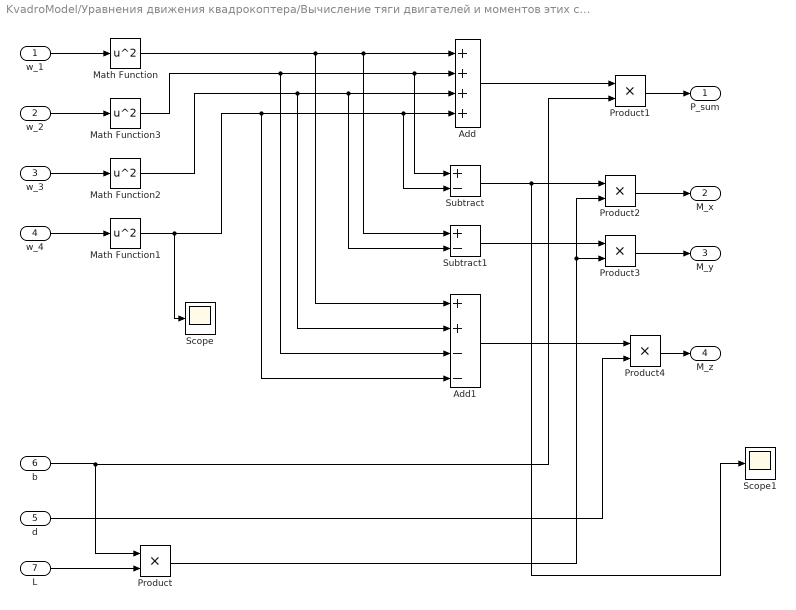
== system KvadroModel/Уравнения движения квадрокоптера/Вычисление тяги двигателей и моментов этих сил ==
  w_1 : Inport
  w_2 : Inport  Port=2
  w_3 : Inport  Port=3
  w_4 : Inport  Port=4
  d : Inport  Port=5
  b : Inport  Port=6
  L : Inport  Port=7
  Add : Sum  Inputs=++++
  Add1 : Sum  Inputs=++--
  Math Function{,1..3} (4 alike) : Math  Operator=square  SaturateOnIntegerOverflow=on
  Product{,1..4} (5 alike) : Product
  Scope : Scope
      settings: YMin=2.5  YMax=42.5  SaveName=ScopeData43
  Scope1 : Scope
      settings: YMin=0.135  YMax=0.205  SaveName=ScopeData45
  Subtract : Sum  Inputs=+-
  Subtract1 : Sum  Inputs=+-
  P_sum : Outport
  M_x : Outport  Port=2
  M_y : Outport  Port=3
  M_z : Outport  Port=4
  wires:
  w_1/1 -> Math Function/1
  w_4/1 -> Math Function1/1
  w_3/1 -> Math Function2/1
  w_2/1 -> Math Function3/1
  Math Function/1 -> Add1/1, Subtract1/1, Add/1
  Math Function3/1 -> Subtract/1, Add/2, Add1/3
  Math Function2/1 -> Subtract1/2, Add/3, Add1/2
  Math Function1/1 -> Scope/1, Add/4, Subtract/2, Add1/4
  b/1 -> Product1/2, Product/1
  L/1 -> Product/2
  Add/1 -> Product1/1
  Product1/1 -> P_sum/1
  Product2/1 -> M_x/1
  Subtract/1 -> Scope1/1, Product2/1
  Subtract1/1 -> Product3/1
  Product/1 -> Product2/2, Product3/2
  Product3/1 -> M_y/1
  Add1/1 -> Product4/1
  d/1 -> Product4/2
  Product4/1 -> M_z/1

== system KvadroModel/Уравнения движения квадрокоптера/Модель сопротивления воздуха (на текущий момент только коэфф.) ==
  Dr : Inport
  DCM : Inport  Port=2
  Gain : Gain  Gain=0.1
  Product : Product  Multiplication=Matrix(*)  RndMeth=Zero
  R : Outport
  wires:
  Dr/1 -> Gain/1
  Product/1 -> R/1
  Gain/1 -> Product/2
  DCM/1 -> Product/1

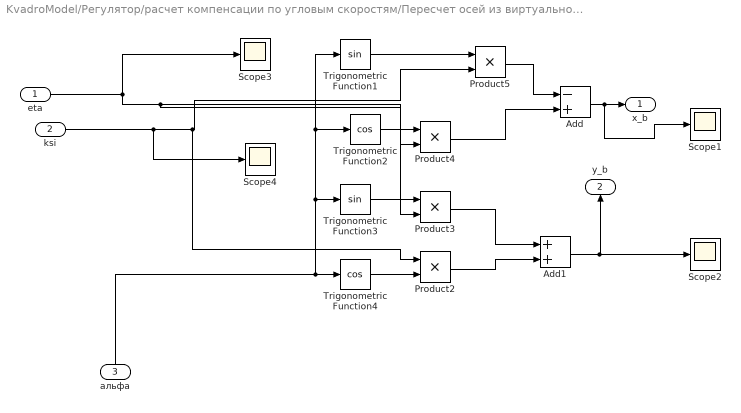
== system KvadroModel/Регулятор/расчет компенсации по угловым скоростям/Пересчет осей из виртуальной в связанную1 ==
  eta : Inport
  ksi : Inport  Port=2
  альфа : Inport  Port=3
  Add : Sum  Inputs=-+
  Add1 : Sum
  Product{2..5} (4 alike) : Product
  Scope{1..4} (4 alike) : Scope
      Scope1 settings: YMin=-3.5  YMax=3.5  SaveName=ScopeData10
      Scope2 settings: YMin=-3.5  YMax=3.5  SaveName=ScopeData11
      Scope3 settings: YMin=-3.5  YMax=3.5  SaveName=ScopeData8
      Scope4 settings: YMin=-3.5  YMax=3.5  SaveName=ScopeData9
  Trigonometric Function1 : Trigonometry
  Trigonometric Function2 : Trigonometry  Operator=cos
  Trigonometric Function3 : Trigonometry
  Trigonometric Function4 : Trigonometry  Operator=cos
  x_b : Outport
  y_b : Outport  Port=2
  wires:
  Trigonometric Function4/1 -> Product2/2
  Trigonometric Function3/1 -> Product3/1
  Trigonometric Function2/1 -> Product4/1
  ksi/1 -> Scope4/1, Product2/1, Product5/2
  eta/1 -> Product3/2, Product4/2, Scope3/1
  Trigonometric Function1/1 -> Product5/1
  альфа/1 -> Trigonometric Function4/1, Trigonometric Function3/1, Trigonometric Function2/1, Trigonometric Function1/1
  Product5/1 -> Add/1
  Product4/1 -> Add/2
  Product3/1 -> Add1/1
  Product2/1 -> Add1/2
  Add1/1 -> Scope2/1, y_b/1
  Add/1 -> Scope1/1, x_b/1

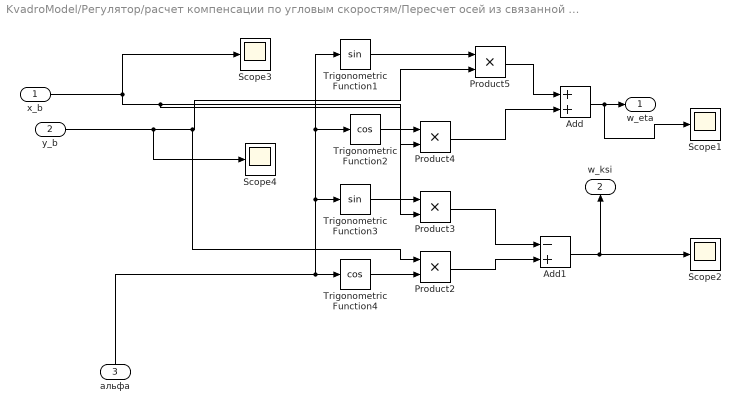
== system KvadroModel/Регулятор/расчет компенсации по угловым скоростям/Пересчет осей из связанной в виртуальную1 ==
  x_b : Inport
  y_b : Inport  Port=2
  альфа : Inport  Port=3
  Add : Sum
  Add1 : Sum  Inputs=-+
  Product{2..5} (4 alike) : Product
  Scope{1..4} (4 alike) : Scope
      Scope1 settings: YMin=-3.5  YMax=3.5  SaveName=ScopeData10
      Scope2 settings: YMin=-3.5  YMax=3.5  SaveName=ScopeData11
      Scope3 settings: YMin=-3.5  YMax=3.5  SaveName=ScopeData8
      Scope4 settings: YMin=-3.5  YMax=3.5  SaveName=ScopeData9
  Trigonometric Function1 : Trigonometry
  Trigonometric Function2 : Trigonometry  Operator=cos
  Trigonometric Function3 : Trigonometry
  Trigonometric Function4 : Trigonometry  Operator=cos
  w_eta : Outport
  w_ksi : Outport  Port=2
  wires:
  Trigonometric Function4/1 -> Product2/2
  Trigonometric Function3/1 -> Product3/1
  Trigonometric Function2/1 -> Product4/1
  y_b/1 -> Scope4/1, Product2/1, Product5/2
  x_b/1 -> Product3/2, Product4/2, Scope3/1
  Trigonometric Function1/1 -> Product5/1
  альфа/1 -> Trigonometric Function4/1, Trigonometric Function3/1, Trigonometric Function2/1, Trigonometric Function1/1
  Product5/1 -> Add/1
  Product4/1 -> Add/2
  Product3/1 -> Add1/1
  Product2/1 -> Add1/2
  Add1/1 -> Scope2/1, w_ksi/1
  Add/1 -> Scope1/1, w_eta/1

== system KvadroModel/Регулятор/расчет компенсации по угловым скоростям плавающего/Пересчет осей обратный1 ==
  x_v : Inport
  y_v : Inport  Port=2
  альфа : Inport  Port=3
  Add : Sum
  Add1 : Sum  Inputs=-+
  Product{2..5} (4 alike) : Product
  Scope1 : Scope
      settings: YMin=-3.5  YMax=3.5  SaveName=ScopeData10
  Scope2 : Scope
      settings: YMin=-3.5  YMax=3.5  SaveName=ScopeData11
  Trigonometric Function1 : Trigonometry  Operator=cos
  Trigonometric Function2 : Trigonometry
  Trigonometric Function3 : Trigonometry
  Trigonometric Function4 : Trigonometry  Operator=cos
  x_b : Outport
  y_b : Outport  Port=2
  wires:
  Add1/1 -> Scope2/1, y_b/1
  Add/1 -> Scope1/1, x_b/1
  Trigonometric Function4/1 -> Product2/2
  Trigonometric Function3/1 -> Product3/1
  Trigonometric Function2/1 -> Product4/1
  y_v/1 -> Product4/2, Product2/1
  Trigonometric Function1/1 -> Product5/1
  альфа/1 -> Trigonometric Function2/1, Trigonometric Function1/1, Trigonometric Function3/1, Trigonometric Function4/1
  Product5/1 -> Add/1
  Product4/1 -> Add/2
  Product3/1 -> Add1/1
  Product2/1 -> Add1/2
  x_v/1 -> Product3/2, Product5/2
